simulink model "linmodel"  (R2025a)
settings: Solver=VariableStepAuto  StartTime=0.0  StopTime=1  RelTol=1e-3
values from neighbouring files (symbols this model uses):
  A = [0 0 0 0 0 1 1 ... (first row only)    [rhs.m]    (also in simulate_sys.m = [mw 0 0 1 -1 0)
  C = eye(length(A))    [determineABK.m]
  D = zeros(length(B), 1)    [determineABK.m]
  k = lqr(A, B, Q, R)    [determineABK.m]
  r = [0;0;0;0]    [determineABK.m]
undefined symbols (not defined in the file or in its folder): B
settings Model: Creator=quintenpienaar  LastModifiedBy=quintenpienaar
settings DataIOCC: SaveOutput=off  SignalLogging=off  DSMLogging=off  SaveTime=off  ReturnWorkspaceOutputs=off

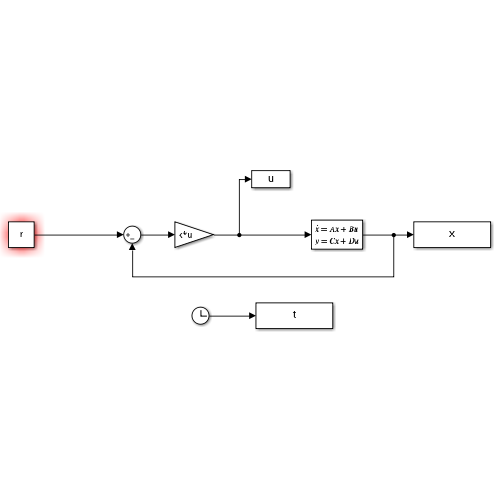
[thumbnail: Simulink's stored preview of the top-level diagram]
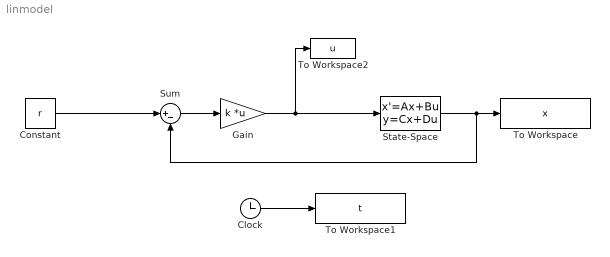
== system linmodel ==
  Clock : Clock
  Constant : Constant  Value=r
  Gain : Gain  Gain=k  Multiplication=Matrix(K*u)
  State-Space : StateSpace  A=A  B=B  C=C  D=D  InitialCondition=0
  Sum : Sum  Inputs=|+-
  To Workspace : ToWorkspace  VariableName=x  SampleTime=-1
      settings: Save2DSignal=2-D array (concatenate along first dimension)
  To Workspace1 : ToWorkspace  VariableName=t  SampleTime=-1
      settings: Save2DSignal=2-D array (concatenate along first dimension)
  To Workspace2 : ToWorkspace  VariableName=u  SampleTime=-1
      settings: Save2DSignal=2-D array (concatenate along first dimension)
  wires:
  State-Space/1 -> Sum/2, To Workspace/1
  Sum/1 -> Gain/1
  Gain/1 -> To Workspace2/1, State-Space/1
  Constant/1 -> Sum/1
  Clock/1 -> To Workspace1/1
